simulink model "realign"  (Simulink 6.2)
settings: Solver=ode45  StartTime=0.0  StopTime=100.0  RelTol=1e-3
libraries: xbsIndex_r3 x17, simulink x6
settings Model: LastModifiedBy=mdexter
settings DebuggingCC: SolverPrmCheckMsg=warning

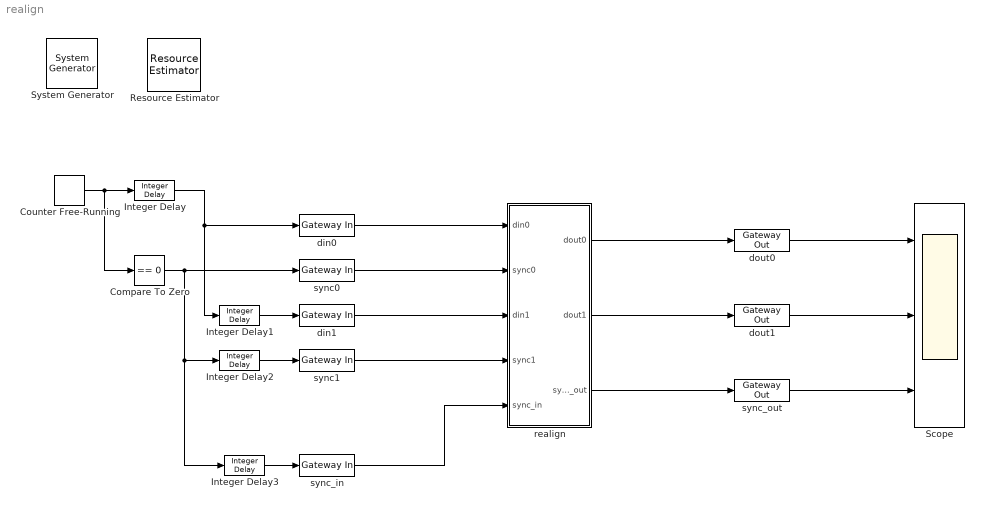
== system realign ==
  " System Generator" : xbsIndex_r3/ System Generator  Tag=genX  xilinxfamily=Virtex2  part=xc2v1000  speed=-4  package=bg575  synthesis_tool=XST  directory=./netlist  testbench=off  simulink_period=1  sysclk_period=100  incr_netlist=off  trim_vbits=Everywhere in SubSystem  dbl_ovrd=According to Block Masks  core_generation=According to Block Masks  run_coregen=off  deprecated_control=off  eval_field=0
      settings: AttributesFormatString=System\nGenerator
  Compare To Zero : simulink/Logic and Bit Operations/Compare To Zero  relop===  LogicOutDataTypeMode=boolean  ZeroCross=off
  Counter Free-Running : simulink/Sources/Counter Free-Running  NumBits=10  tsamp=-1
  Integer Delay : simulink/Discrete/Integer Delay  vinit=0.0  samptime=-1  NumDelays=1
  Integer Delay1 : simulink/Discrete/Integer Delay  vinit=0.0  samptime=-1  NumDelays=10
  Integer Delay2 : simulink/Discrete/Integer Delay  vinit=0.0  samptime=-1  NumDelays=10
  Integer Delay3 : simulink/Discrete/Integer Delay  vinit=0.0  samptime=-1  NumDelays=32
  Resource Estimator : xbsIndex_r3/Resource Estimator  Tag=resEstTag  xl_estimator_area=[398 26 0 780 260 0 0]  xl_use_estimator_area=off  simulink_period=1  mrp_directory=./netlist
      settings: AttributesFormatString=Resource\nEstimator
  Scope : Scope  NumInputPorts=3
      settings: YMin=-5~-5~-5  YMax=5~5~5
  din0 : xbsIndex_r3/Gateway In  arith_type=Unsigned  n_bits=64  bin_pt=0  quantization=Truncate  overflow=Wrap  period=1  timing_constraint=None  locs_specified=off  LOCs={}  needs_fixed_name=off  dbl_ovrd=off  show_param=on
      settings: xl_area=[0 0 0 0 64 0 0]
  din1 : xbsIndex_r3/Gateway In  arith_type=Unsigned  n_bits=64  bin_pt=0  quantization=Truncate  overflow=Wrap  period=1  timing_constraint=None  locs_specified=off  LOCs={}  needs_fixed_name=off  dbl_ovrd=off  show_param=on
      settings: xl_area=[0 0 0 0 64 0 0]
  dout0 : xbsIndex_r3/Gateway Out  output_type=Double  nbits=8  bin_pt=6  arith_type=Boolean  quantization=Truncate  overflow=Wrap  hdl_port=on  timing_constraint=None  locs_specified=off  LOCs={}  needs_fixed_name=off  show_param=off
      settings: xl_area=[0 0 0 0 64 0 0]
  dout1 : xbsIndex_r3/Gateway Out  output_type=Double  nbits=8  bin_pt=6  arith_type=Boolean  quantization=Truncate  overflow=Wrap  hdl_port=on  timing_constraint=None  locs_specified=off  LOCs={}  needs_fixed_name=off  show_param=off
      settings: xl_area=[0 0 0 0 64 0 0]
  realign : Subsystem
  sync0 : xbsIndex_r3/Gateway In  arith_type=Boolean  n_bits=64  bin_pt=0  quantization=Truncate  overflow=Wrap  period=1  timing_constraint=None  locs_specified=off  LOCs={}  needs_fixed_name=off  dbl_ovrd=off  show_param=on
      settings: xl_area=[0 0 0 0 1 0 0]
  sync1 : xbsIndex_r3/Gateway In  arith_type=Boolean  n_bits=64  bin_pt=0  quantization=Truncate  overflow=Wrap  period=1  timing_constraint=None  locs_specified=off  LOCs={}  needs_fixed_name=off  dbl_ovrd=off  show_param=on
      settings: xl_area=[0 0 0 0 1 0 0]
  sync_in : xbsIndex_r3/Gateway In  arith_type=Boolean  n_bits=64  bin_pt=0  quantization=Truncate  overflow=Wrap  period=1  timing_constraint=None  locs_specified=off  LOCs={}  needs_fixed_name=off  dbl_ovrd=off  show_param=on
      settings: xl_area=[0 0 0 0 1 0 0]
  sync_out : xbsIndex_r3/Gateway Out  output_type=Double  nbits=8  bin_pt=6  arith_type=Boolean  quantization=Truncate  overflow=Wrap  hdl_port=on  timing_constraint=None  locs_specified=off  LOCs={}  needs_fixed_name=off  show_param=off
      settings: xl_area=[0 0 0 0 1 0 0]
  wires:
  din0/1 -> realign/1(din0)
  sync0/1 -> realign/2(sync0)
  realign/1(dout0) -> dout0/1
  din1/1 -> realign/3(din1)
  sync1/1 -> realign/4(sync1)
  realign/2(dout1) -> dout1/1
  sync_in/1 -> realign/5(sync_in)
  Counter Free-Running/1 -> Compare To Zero/1, Integer Delay/1
  Integer Delay/1 -> din0/1, Integer Delay1/1
  Compare To Zero/1 -> sync0/1, Integer Delay2/1, Integer Delay3/1
  Integer Delay1/1 -> din1/1
  Integer Delay2/1 -> sync1/1
  Integer Delay3/1 -> sync_in/1
  dout0/1 -> Scope/1
  dout1/1 -> Scope/2
  sync_out/1 -> Scope/3
  realign/3(sync_out) -> sync_out/1

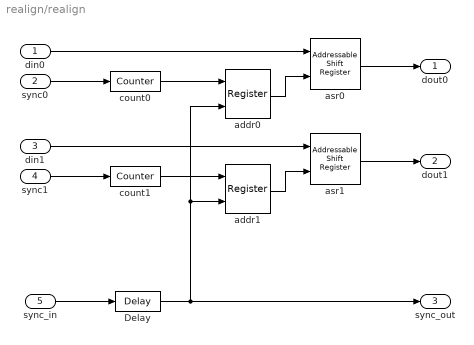
== system realign/realign ==
  din0 : Inport  Port=1  LatchInput=off
  sync0 : Inport  Port=2  LatchInput=off
  din1 : Inport  Port=3  LatchInput=off
  sync1 : Inport  Port=4  LatchInput=off
  sync_in : Inport  Port=5  LatchInput=off
  Delay : xbsIndex_r3/Delay  latency=1  reg_retiming=off  explicit_period=off  period=1  en=off  accept_only_valid=off  init_zero=on  dbl_ovrd=off  show_param=off
      settings: xl_area=[1 1 0 0 0 0 0]
  addr0 : xbsIndex_r3/Register  init=0  reg_only_valid=off  explicit_period=off  period=1  rst=off  en=on  out_en=off  dbl_ovrd=off  show_param=on
      settings: xl_area=[3 6 0 0 0 0 0]
  addr1 : xbsIndex_r3/Register  init=0  reg_only_valid=off  explicit_period=off  period=1  rst=off  en=on  out_en=off  dbl_ovrd=off  show_param=on
      settings: xl_area=[3 6 0 0 0 0 0]
  asr0 : xbsIndex_r3/Addressable Shift Register  infer_latency=on  depth=2  initVector=[0]  explicit_period=off  period=1  accept_only_valid=off  en=off  dbl_ovrd=off  show_param=on  use_rpm=on  gen_core=off
      settings: xl_area=[192 0 0 384 0 0 0]
  asr1 : xbsIndex_r3/Addressable Shift Register  infer_latency=on  depth=2  initVector=[0]  explicit_period=off  period=1  accept_only_valid=off  en=off  dbl_ovrd=off  show_param=on  use_rpm=on  gen_core=off
      settings: xl_area=[192 0 0 384 0 0 0]
  count0 : xbsIndex_r3/Counter  cnt_type=Free Running  n_bits=6  bin_pt=0  arith_type=Unsigned  start_count=0  cnt_to=Inf  cnt_by_val=1  operation=Up  explicit_period=off  period=1  load_pin=off  rst=on  en=off  dbl_ovrd=off  show_param=on  use_rpm=on  gen_core=off
      settings: xl_area=[3 6 0 6 0 0 0]
  count1 : xbsIndex_r3/Counter  cnt_type=Free Running  n_bits=6  bin_pt=0  arith_type=Unsigned  start_count=0  cnt_to=Inf  cnt_by_val=1  operation=Up  explicit_period=off  period=1  load_pin=off  rst=on  en=off  dbl_ovrd=off  show_param=on  use_rpm=on  gen_core=off
      settings: xl_area=[3 6 0 6 0 0 0]
  dout0 : Outport
  dout1 : Outport  Port=2
  sync_out : Outport  Port=3
  wires:
  count0/1 -> addr0/1
  addr0/1 -> asr0/2
  count1/1 -> addr1/1
  addr1/1 -> asr1/2
  Delay/1 -> addr1/2, addr0/2, sync_out/1
  din0/1 -> asr0/1
  asr0/1 -> dout0/1
  sync0/1 -> count0/1
  din1/1 -> asr1/1
  asr1/1 -> dout1/1
  sync1/1 -> count1/1
  sync_in/1 -> Delay/1
